simulink model "mpc_dcmotor_simulink_S"  (R2018b)
settings: Solver=VariableStepAuto  StartTime=0  StopTime=15  RelTol=1e-3
values from neighbouring files (symbols this model uses):
  k = 1    [mpc_dcmotor.m]    (also in mpc_dcmotor_Tmpc.m; mpc_dcmotor_simulink.m)
  maxIter = 100    [mpc_dcmotor.m]    (also in mpc_dcmotor_Tmpc.m = 50; mpc_dcmotor_simulink.m = 50; mpc_quadcopter.m = 1000; mpc_unicycle.m = 300)
  mu0 = 1e-3    (= 0.001)    [mpc_dcmotor.m]    (also in mpc_dcmotor_Tmpc.m = 1; mpc_dcmotor_simulink.m = 1; mpc_quadcopter.m; mpc_unicycle.m = 1)
  p = -2    [mpc_dcmotor.m]    (also in mpc_dcmotor_Tmpc.m = 2; mpc_dcmotor_simulink.m = 2; mpc_quadcopter.m = ppval(cs,t))
  refmax = .35    (= 0.35)    [mpc_dcmotor_Tmpc.m]    (also in mpc_dcmotor_simulink.m)
  refomega = .5    (= 0.5)    [mpc_dcmotor_Tmpc.m]    (also in mpc_dcmotor_simulink.m)
  saveIter = -1    [mpc_dcmotor.m]    (also in mpc_dcmotor_Tmpc.m = false; mpc_dcmotor_simulink.m = 0; mpc_quadcopter.m; mpc_unicycle.m)
  T = 30    [mpc_dcmotor.m]    (also in mpc_dcmotor_Tmpc.m; mpc_dcmotor_simulink.m; mpc_quadcopter.m = 100; mpc_unicycle.m = 200)
  Ts = .1    (= 0.1)    [mpc_dcmotor.m]    (also in mpc_dcmotor_Tmpc.m; mpc_dcmotor_simulink.m; mpc_quadcopter.m = 0.02; mpc_unicycle.m = 0.01)
  u_cold = .1*randn(nu,T)    [mpc_dcmotor_simulink.m]
  umax = 1    [mpc_dcmotor_simulink.m]
  x1_cold = .1*randn(nx,T)    [mpc_dcmotor_simulink.m]
  xmax = [.4;.3]    [mpc_dcmotor_Tmpc.m]    (also in mpc_dcmotor_simulink.m)
settings Model: Creator=hespanha  LastModifiedBy=hespanha

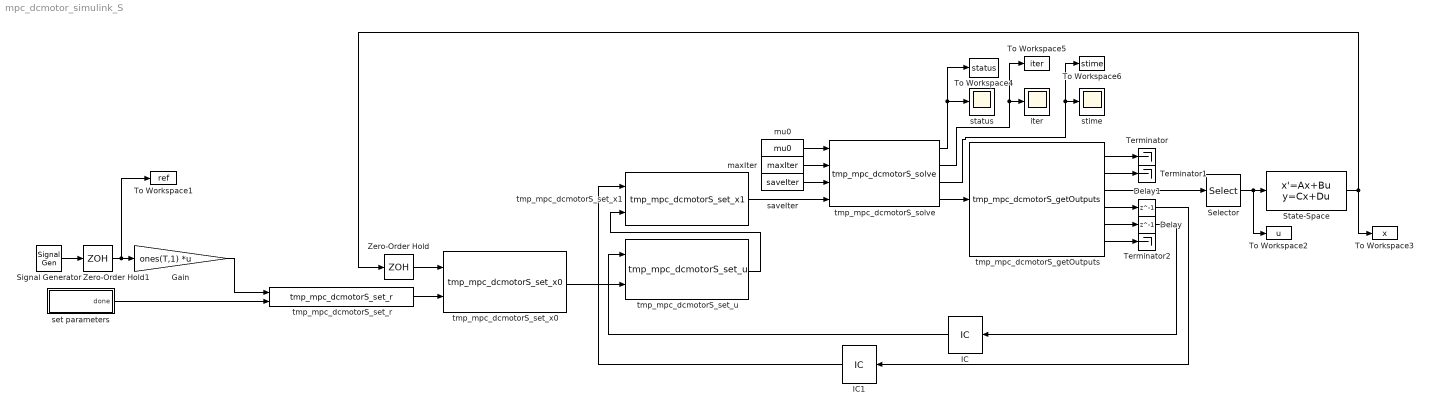
== system mpc_dcmotor_simulink_S ==
  Delay : Delay  DelayLength=1
  Delay1 : Delay  DelayLength=1
  Gain : Gain  Gain=ones(T,1)  Multiplication=Matrix(K*u)
  IC : InitialCondition  Value=u_cold
  IC1 : InitialCondition  Value=x1_cold
  Selector : Selector  NumberOfDimensions=2  InputPortWidth=3  IndexOptions=Select all,Index vector (dialog)  Indices=[1 3],1  OutputSizes=1,1
  Signal Generator : SignalGenerator  WaveForm=square  Amplitude=refmax  Frequency=refomega  Units=rad/sec
  State-Space : StateSpace  A=[0,1;0,p]  B=[0;k]  C=eye(2)  D=zeros(2,1)  InitialCondition=[.2;.2]  ContinuousStateAttributes={'theta','x2'}
  Terminator : Terminator
  Terminator1 : Terminator
  Terminator2 : Terminator
  To Workspace1 : ToWorkspace  VariableName=ref  SaveFormat=Structure With Time  SampleTime=-1
  To Workspace2 : ToWorkspace  VariableName=u  SaveFormat=Structure With Time  SampleTime=-1
      settings: Save2DSignal=2-D array (concatenate along first dimension)
  To Workspace3 : ToWorkspace  VariableName=x  SaveFormat=Structure With Time  SampleTime=-1
  To Workspace4 : ToWorkspace  VariableName=status  SaveFormat=Structure With Time  SampleTime=-1
      settings: Save2DSignal=2-D array (concatenate along first dimension)
  To Workspace5 : ToWorkspace  VariableName=iter  SaveFormat=Structure With Time  SampleTime=-1
      settings: Save2DSignal=2-D array (concatenate along first dimension)
  To Workspace6 : ToWorkspace  VariableName=stime  SaveFormat=Structure With Time  SampleTime=-1
      settings: Save2DSignal=2-D array (concatenate along first dimension)
  Zero-Order Hold : ZeroOrderHold  SampleTime=Ts
  Zero-Order Hold1 : ZeroOrderHold  SampleTime=Ts
  iter : Scope
  maxIter : Constant  Value=maxIter  OutDataTypeStr=int32
  mu0 : Constant  Value=mu0
  saveIter : Constant  Value=saveIter  OutDataTypeStr=int32
  set parameters : Subsystem
  status : Scope
  stime : Scope
  tmp_mpc_dcmotorS_getOutputs : S-Function  FunctionName=tmp_mpc_dcmotorS_getOutputs  SFunctionDeploymentMode=off  EnableBusSupport=off
  tmp_mpc_dcmotorS_set_r : S-Function  FunctionName=tmp_mpc_dcmotorS_set_r  SFunctionDeploymentMode=off  EnableBusSupport=off
  tmp_mpc_dcmotorS_set_u : S-Function  FunctionName=tmp_mpc_dcmotorS_set_u  SFunctionDeploymentMode=off  EnableBusSupport=off
  tmp_mpc_dcmotorS_set_x0 : S-Function  FunctionName=tmp_mpc_dcmotorS_set_x0  SFunctionDeploymentMode=off  EnableBusSupport=off
  tmp_mpc_dcmotorS_set_x1 : S-Function  FunctionName=tmp_mpc_dcmotorS_set_x1  SFunctionDeploymentMode=off  EnableBusSupport=off
  tmp_mpc_dcmotorS_solve : S-Function  FunctionName=tmp_mpc_dcmotorS_solve  SFunctionDeploymentMode=off  EnableBusSupport=off
  wires:
  tmp_mpc_dcmotorS_getOutputs/1 -> Terminator/1
  tmp_mpc_dcmotorS_getOutputs/2 -> Terminator1/1
  tmp_mpc_dcmotorS_getOutputs/5 -> Delay/1
  tmp_mpc_dcmotorS_getOutputs/4 -> Delay1/1
  tmp_mpc_dcmotorS_getOutputs/6 -> Terminator2/1
  tmp_mpc_dcmotorS_getOutputs/3 -> Selector/1
  Selector/1 -> To Workspace2/1, State-Space/1
  tmp_mpc_dcmotorS_solve/4 -> tmp_mpc_dcmotorS_getOutputs/1
  tmp_mpc_dcmotorS_solve/2 -> To Workspace5/1, iter/1
  tmp_mpc_dcmotorS_solve/1 -> To Workspace4/1, status/1
  tmp_mpc_dcmotorS_solve/3 -> To Workspace6/1, stime/1
  tmp_mpc_dcmotorS_set_x0/1 -> tmp_mpc_dcmotorS_set_u/2
  mu0/1 -> tmp_mpc_dcmotorS_solve/1
  maxIter/1 -> tmp_mpc_dcmotorS_solve/2
  saveIter/1 -> tmp_mpc_dcmotorS_solve/3
  Delay1/1 -> IC1/1
  Delay/1 -> IC/1
  tmp_mpc_dcmotorS_set_u/1 -> tmp_mpc_dcmotorS_set_x1/2
  tmp_mpc_dcmotorS_set_x1/1 -> tmp_mpc_dcmotorS_solve/4
  State-Space/1 -> To Workspace3/1, Zero-Order Hold/1
  Zero-Order Hold/1 -> tmp_mpc_dcmotorS_set_x0/1
  IC/1 -> tmp_mpc_dcmotorS_set_u/1
  IC1/1 -> tmp_mpc_dcmotorS_set_x1/1
  tmp_mpc_dcmotorS_set_r/1 -> tmp_mpc_dcmotorS_set_x0/2
  set parameters/1(done) -> tmp_mpc_dcmotorS_set_r/2
  Signal Generator/1 -> Zero-Order Hold1/1
  Gain/1 -> tmp_mpc_dcmotorS_set_r/1
  Zero-Order Hold1/1 -> To Workspace1/1, Gain/1

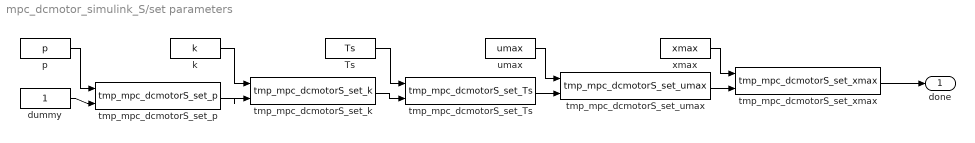
== system mpc_dcmotor_simulink_S/set parameters ==
  Ts : Constant  Value=Ts
  "dummy " : Constant
  k : Constant  Value=k
  "p " : Constant  Value=p
  tmp_mpc_dcmotorS_set_Ts : S-Function  FunctionName=tmp_mpc_dcmotorS_set_Ts  SFunctionDeploymentMode=off  EnableBusSupport=off
  tmp_mpc_dcmotorS_set_k : S-Function  FunctionName=tmp_mpc_dcmotorS_set_k  SFunctionDeploymentMode=off  EnableBusSupport=off
  tmp_mpc_dcmotorS_set_p : S-Function  FunctionName=tmp_mpc_dcmotorS_set_p  SFunctionDeploymentMode=off  EnableBusSupport=off
  tmp_mpc_dcmotorS_set_umax : S-Function  FunctionName=tmp_mpc_dcmotorS_set_umax  SFunctionDeploymentMode=off  EnableBusSupport=off
  tmp_mpc_dcmotorS_set_xmax : S-Function  FunctionName=tmp_mpc_dcmotorS_set_xmax  SFunctionDeploymentMode=off  EnableBusSupport=off
  umax : Constant  Value=umax
  xmax : Constant  Value=xmax
  done : Outport
  wires:
  "dummy "/1 -> tmp_mpc_dcmotorS_set_p/2
  Ts/1 -> tmp_mpc_dcmotorS_set_Ts/1
  tmp_mpc_dcmotorS_set_xmax/1 -> done/1
  "p "/1 -> tmp_mpc_dcmotorS_set_p/1
  xmax/1 -> tmp_mpc_dcmotorS_set_xmax/1
  tmp_mpc_dcmotorS_set_umax/1 -> tmp_mpc_dcmotorS_set_xmax/2
  tmp_mpc_dcmotorS_set_Ts/1 -> tmp_mpc_dcmotorS_set_umax/2
  k/1 -> tmp_mpc_dcmotorS_set_k/1
  tmp_mpc_dcmotorS_set_k/1 -> tmp_mpc_dcmotorS_set_Ts/2
  umax/1 -> tmp_mpc_dcmotorS_set_umax/1
  tmp_mpc_dcmotorS_set_p/1 -> tmp_mpc_dcmotorS_set_k/2
